simulink model "Lab6_dyskretny_2015a"  (R2015a)
settings: Solver=ode45  SolverMode=SingleTasking  StartTime=0.0  StopTime=10.0  FixedStep=0.01  RelTol=1e-3
values from neighbouring files (symbols this model uses):
  h = bodeplot(K)    [Lab1.m]    (also in Lab5.m = nyquistplot(K0); Lab6.m = 0.5*Tmax)
libraries: cstblocks x2
settings Model: CovMetricSettings=dwe  CovHtmlReporting=off  covSaveCumulativeToWorkspaceVar=off  CovSaveSingleToWorkspaceVar=off  CovExternalEMLEnable=on  Creator=ishiguro  LastModifiedBy=ishiguro
settings DataIOCC: LimitDataPoints=off  SaveFormat=Dataset  TimeSaveName=tout_dysk
settings DebuggingCC: SFUnexpectedBacktrackingDiag=error  SFNoUnconditionalDefaultTransitionDiag=error
settings HardwareCC: ProdBitPerPointer=64  ProdLargestAtomicFloat=Float  ProdIntDivRoundTo=Zero  ProdEndianess=LittleEndian  ProdHWDeviceType=Specified
settings ModelReferenceCC: PropagateSignalLabelsOutOfModel=on
settings GRTTargetCC: TargetLangStandard=C99 (ISO)  GeneratePreprocessorConditionals=Use local settings

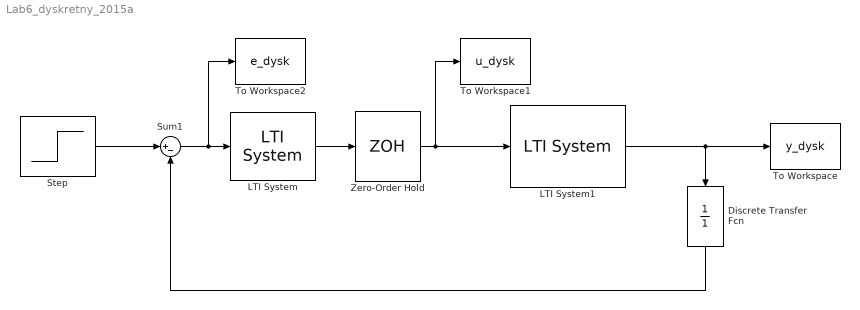
== system Lab6_dyskretny_2015a ==
  Discrete Transfer Fcn : DiscreteTransferFcn  Denominator=[1]  SampleTime=h
  LTI System : cstblocks/LTI System  sys=Kr  IC=[]
  LTI System1 : cstblocks/LTI System  sys=K  IC=[]
  Step : Step  Time=0  SampleTime=0
  Sum1 : Sum  Inputs=|+-
  To Workspace : ToWorkspace  VariableName=y_dysk  SampleTime=-1
  To Workspace1 : ToWorkspace  VariableName=u_dysk  SampleTime=-1
  To Workspace2 : ToWorkspace  VariableName=e_dysk  SampleTime=-1
  Zero-Order Hold : ZeroOrderHold  SampleTime=h
  wires:
  Sum1/1 -> To Workspace2/1, LTI System/1
  Step/1 -> Sum1/1
  LTI System1/1 -> Discrete Transfer Fcn/1, To Workspace/1
  Discrete Transfer Fcn/1 -> Sum1/2
  LTI System/1 -> Zero-Order Hold/1
  Zero-Order Hold/1 -> To Workspace1/1, LTI System1/1
